simulink model "open_loop_lateral_dyn_2023b"  (R2023b)
settings: Solver=VariableStepAuto  StartTime=0.0  StopTime=Ts  RelTol=1e-3
values from neighbouring files (symbols this model uses):
  A = [0 1 0 0 ... (first row only)    [system_mat.m]
  af = 1.3    [Gain.m]    (also in Init.m; beta_vs_delta_tf.m; r_vs_delta_tf.m; system_mat.m)
  ar = 1.5    [Gain.m]    (also in Init.m; beta_vs_delta_tf.m; r_vs_delta_tf.m; system_mat.m)
  B = [B1 B2]    [system_mat.m]
  CF = 2*6*1e4    (= 120000)    [Gain.m]    (also in Init.m; beta_vs_delta_tf.m; r_vs_delta_tf.m; system_mat.m)
  CR = 2*5.7*1e4    (= 114000)    [Gain.m]    (also in Init.m; beta_vs_delta_tf.m; r_vs_delta_tf.m; system_mat.m)
  delay_return = 13+delay    (= 14)    [Init.m]
  delta_max = 25    [Gain.m]    (also in Init.m)
  dvol_drift1 = dvol_drift(1)    [Init.m]
  dvol_drift2 = dvol_drift(2)    [Init.m]
  dvol_drift3 = dvol_drift(3)    [Init.m]
  K = (m/L)*(CR*ar-(CF*af))/(CF*CR)    (= 0.000616776315789)    [Gain.m]    (also in Init.m = place(A,B(:,1),p); Poles.m = acker(A, B(:,1), P(i,:)))
  L = af+ar    (= 2.8)    [Gain.m]    (also in Init.m)
  m = 1575    [Gain.m]    (also in Init.m; beta_vs_delta_tf.m; r_vs_delta_tf.m; system_mat.m)
  sel_man = 1    [Init.m]
  t_drift_cs_1 = 5*1+3*0    (= 5)    [Init.m]
  t_drift_cs_2 = t_drift_cs_1*2    (= 10)    [Init.m]
  tau_s = 15    [Gain.m]    (also in Init.m)
  Vx = vv(i)    [Gain.m]    (also in Init.m = 22.2222222222; Transfer_functions.m = 33.3333333333)
libraries: simulink_extras x4, simulink x4
settings Model: Creator=soffy  LastModifiedBy=Martina
settings DataIOCC: ReturnWorkspaceOutputs=off

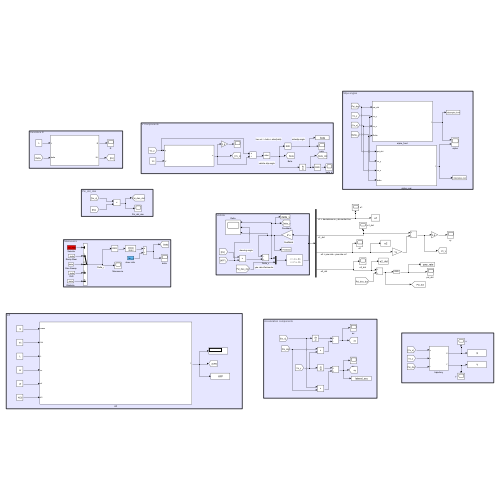
[thumbnail: Simulink's stored preview of the top-level diagram]
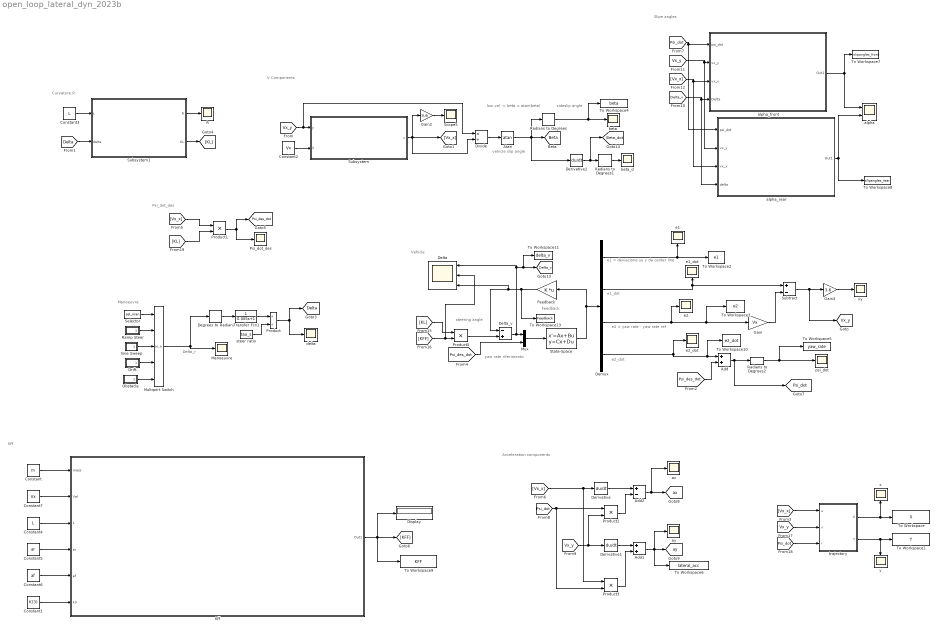
== system open_loop_lateral_dyn_2023b ==
  note: Feedback
  note: Delta_r
  note: Psi_dot_des
  note: sideslip angle
  note: Manoeuvre
  note: Vehicle
  note: Acceleration components
  note: Kff
  note: Curvature R
  note: vehicle slip angle
  note: low vel -> beta = atan(beta)
  note: V Components
  note: e2_dot
  note: e1_dot
  note: e2 = yaw rate - yaw rate ref
  note: e1 = deviazione su y da center line
  note: yaw rate riferimento
  note: steering angle
  note: Slipe angles
  Add : Sum
  Add1 : Sum
  Add2 : Sum  Inputs=+-
  Atan : Trigonometry  Operator=atan
  Constant : Constant  Value=m
  Constant1 : Constant  Value=K(3)
  Constant2 : Constant  Value=Vx
  Constant3 : Constant  Value=L
  Constant4 : Constant  Value=L
  Constant5 : Constant  Value=ar
  Constant6 : Constant  Value=af
  Constant7 : Constant  Value=Vx
  Degrees to Radians : simulink_extras/Transformations/Degrees to Radians
  Delta : Scope  NumInputPorts=3
  Delta_v : Sum  Inputs=-+
  Demux : Demux
  Derivative : Derivative
  Derivative1 : Derivative
  Derivative2 : Derivative
  Display : Display
  Divide : Product  Inputs=*/
  Drift : Subsystem
  Feedback : Gain  Gain=K  Multiplication=Matrix(K*u)
  Gain : Gain  Gain=Vx
  Gain2 : Gain  Gain=3.6
  Gain3 : Gain  Gain=3.6
  Kff : Subsystem
  Manoeuvre : Scope
  Multiport Switch : MultiPortSwitch  Inputs=4  SaturateOnIntegerOverflow=off  InputSameDT=off
  Mux : Mux  Inputs=2
  Obstacle : Subsystem
  Product : Product  Inputs=*/  RndMeth=Zero
  Product{1..3,5} (4 alike) : Product
  Psi_dot_des : Scope
  R : Scope
  Radians to Degrees : simulink_extras/Transformations/Radians to Degrees
  Radians to Degrees1 : simulink_extras/Transformations/Radians to Degrees
  Radians to Degrees2 : simulink_extras/Transformations/Radians to Degrees
  Ramp Steer : Subsystem
  Scope5 : Scope
  Selector : Constant  Value=sel_man
  Sine Sweep : Subsystem
  State-Space : StateSpace  A=A  B=B  C=eye(4)  D=zeros(4,2)  InitialCondition=0
  Subsystem : Subsystem
  Subsystem1 : Subsystem
  Subtract : Sum  Inputs=+-
  To Workspace : ToWorkspace  VariableName=X  SaveFormat=Timeseries  SampleTime=-1
  To Workspace1 : ToWorkspace  VariableName=Y  SaveFormat=Timeseries  SampleTime=-1
  To Workspace10 : ToWorkspace  VariableName=e2_dot  SaveFormat=Timeseries  SampleTime=-1
  To Workspace11 : ToWorkspace  VariableName=delta_v  SaveFormat=Timeseries  SampleTime=-1
  To Workspace13 : ToWorkspace  VariableName=Feedback  SaveFormat=Timeseries  SampleTime=-1
  To Workspace2 : ToWorkspace  VariableName=e1  SaveFormat=Timeseries  SampleTime=-1
  To Workspace3 : ToWorkspace  VariableName=e2  SaveFormat=Timeseries  SampleTime=-1
  To Workspace4 : ToWorkspace  VariableName=beta  SaveFormat=Timeseries  SampleTime=-1
  To Workspace5 : ToWorkspace  VariableName=yaw_rate  SaveFormat=Timeseries  SampleTime=-1
  To Workspace6 : ToWorkspace  VariableName=lateral_acc  SaveFormat=Timeseries  SampleTime=-1
  To Workspace7 : ToWorkspace  VariableName=slipangles_front  SaveFormat=Timeseries  SampleTime=-1
  To Workspace8 : ToWorkspace  VariableName=slipangles_rear  SaveFormat=Timeseries  SampleTime=-1
  To Workspace9 : ToWorkspace  VariableName=KFF  SaveFormat=Timeseries  SampleTime=-1
  Transfer Fcn1 : TransferFcn  Denominator=[0.005 1]
  alpha : Scope  NumInputPorts=2
  alpha_front : Subsystem
  alpha_rear : Subsystem
  ax : Scope
  ay : Scope
  beta : Scope
  beta_d : Scope
  delta : Scope
  e1 : Scope
  e1_dot : Scope
  e2 : Scope
  e2_dot : Scope
  "psi_dot " : Scope
  "steer ratio " : Constant  Value=tau_s
  trajectory : Subsystem
  vy : Scope
  x : Scope
  y : Scope
  tag scope: Beta=global, Beta_dot=global, Delta=global, Delta_v=global, Psi_des_dot=global, Psi_dot=global, Vx_y=global, ax=global, ay=global
  wires:
  Mux/1 -> State-Space/1
  State-Space/1 -> Feedback/1, Demux/1
  Demux/1 -> To Workspace2/1, e1/1
  Demux/2 -> e1_dot/1, Subtract/1
  Demux/3 -> To Workspace3/1, Gain/1, e2/1
  Demux/4 -> e2_dot/1, To Workspace10/1, Add/1
  Degrees to Radians/1 -> Transfer Fcn1/1
  Transfer Fcn1/1 -> Product/1
  "steer ratio "/1 -> Product/2
  Product/1 -> [Delta], delta/1
  Gain/1 -> Subtract/2
  Subtract/1 -> Gain3/1, [Vx_y]
  Add/1 -> [Psi_dot], Radians to Degrees2/1
  Radians to Degrees2/1 -> To Workspace5/1, "psi_dot "/1
  Subsystem/1(x) -> Gain2/1, [Vx_x], Divide/2
  [Vx_y] -> Divide/1, Subsystem/1(y)
  Constant2/1 -> Subsystem/2(V)
  Constant3/1 -> Subsystem1/1(L)
  [Delta] -> Subsystem1/2(delta)
  Subsystem1/2(KL) -> [KL]
  Kff/1(Out1) -> To Workspace9/1, Display/1, [KFF]
  Constant/1 -> Kff/1(mass)
  Constant7/1 -> Kff/2(Vel)
  Constant4/1 -> Kff/3(L)
  Constant5/1 -> Kff/4(ar)
  Constant6/1 -> Kff/5(af)
  [Psi_des_dot] -> Add/2
  [Psi_des_dot] -> Mux/2
  Divide/1 -> Atan/1
  [Vx_x] -> Product1/1
  Product1/1 -> [Psi_des_dot], Psi_dot_des/1
  Atan/1 -> Radians to Degrees/1, Derivative2/1, [Beta]
  [Vx_x] -> Product3/1, Derivative/1
  Add1/1 -> To Workspace6/1, [ay], ay/1
  [Vx_y] -> Product2/2, Derivative1/1
  Derivative1/1 -> Add1/1
  Derivative/1 -> Add2/1
  [Psi_dot] -> Product3/2, Product2/1
  Product2/1 -> Add2/2
  Product3/1 -> Add1/2
  Add2/1 -> ax/1, [ax]
  alpha_front/1(Out1) -> To Workspace7/1, alpha/1
  [Vx_x] -> alpha_rear/3(vx_x), alpha_front/3(vx_x)
  [Delta_v] -> alpha_rear/4(delta), alpha_front/4(Delta)
  [Psi_dot] -> alpha_rear/1(psi_dot), alpha_front/1(psi_dot)
  [Vx_y] -> alpha_rear/2(vx_y), alpha_front/2(vx_y)
  alpha_rear/1(Out1) -> To Workspace8/1, alpha/2
  Delta_v/1 -> To Workspace11/1, [Delta_v], Delta/1, Mux/1
  Feedback/1 -> Delta_v/1, Delta/3, To Workspace13/1
  Product5/1 -> Delta_v/2
  [KFF] -> Delta/2, Product5/2
  [KL] -> Product5/1
  Constant1/1 -> Kff/6(k3)
  Gain2/1 -> Scope5/1
  Gain3/1 -> vy/1
  Derivative2/1 -> Radians to Degrees1/1, [Beta_dot]
  [Vx_x] -> trajectory/1(u)
  [Vx_y] -> trajectory/2(v)
  trajectory/1(X) -> To Workspace/1, x/1
  trajectory/2(Y) -> To Workspace1/1, y/1
  [Psi_dot] -> trajectory/3(r)
  Radians to Degrees1/1 -> beta_d/1
  Radians to Degrees/1 -> To Workspace4/1, beta/1
  Selector/1 -> Multiport Switch/1
  Ramp Steer/1(delta) -> Multiport Switch/2
  Sine Sweep/1(delta) -> Multiport Switch/3
  Drift/1(delta) -> Multiport Switch/4
  Multiport Switch/1 -> Degrees to Radians/1, Manoeuvre/1
  [KL] -> Product1/2
  Subsystem1/1(R) -> R/1
  Obstacle/1(delta) -> Multiport Switch/5

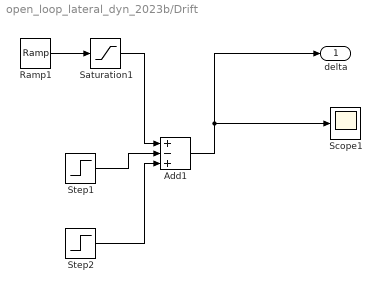
== system open_loop_lateral_dyn_2023b/Drift ==
  Add1 : Sum  Inputs=+-+
  Ramp1 : simulink/Sources/Ramp  slope=400  start=1  InitialOutput=0
  Saturation1 : Saturate  UpperLimit=dvol_drift1  LowerLimit=0
  Scope1 : Scope
  Step1 : Step  Time=t_drift_cs_1  After=dvol_drift2  SampleTime=0
  Step2 : Step  Time=t_drift_cs_2  After=dvol_drift3  SampleTime=0
  delta : Outport  VectorParamsAs1DForOutWhenUnconnected=off
  wires:
  Step2/1 -> Add1/3
  Saturation1/1 -> Add1/1
  Add1/1 -> delta/1, Scope1/1
  Step1/1 -> Add1/2
  Ramp1/1 -> Saturation1/1

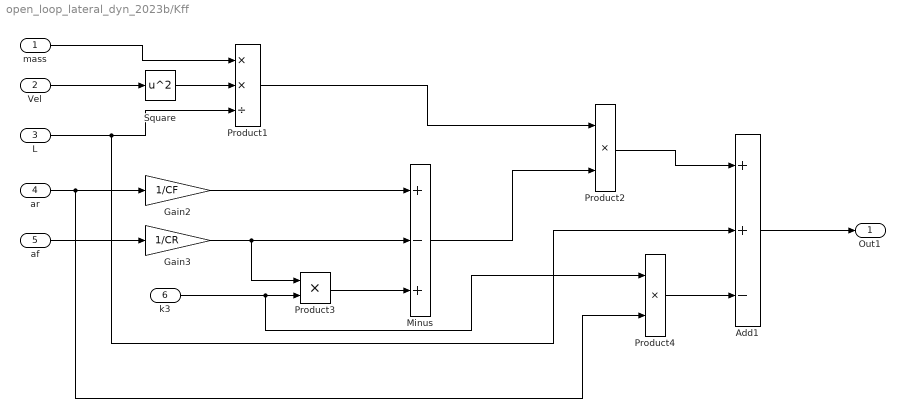
== system open_loop_lateral_dyn_2023b/Kff ==
  mass : Inport
  Vel : Inport  Port=2
  L : Inport  Port=3
  ar : Inport  Port=4
  af : Inport  Port=5
  k3 : Inport  Port=6
  Add1 : Sum  Inputs=++-
  Gain2 : Gain  Gain=1/CF
  Gain3 : Gain  Gain=1/CR
  Minus : Sum  Inputs=+-+
  Product1 : Product  Inputs=**/
  Product2 : Product
  Product3 : Product
  Product4 : Product
  Square : Math  Operator=square
  Out1 : Outport
  wires:
  Product1/1 -> Product2/1
  Product2/1 -> Add1/1
  Gain3/1 -> Minus/2, Product3/1
  Square/1 -> Product1/2
  Product4/1 -> Add1/3
  Product3/1 -> Minus/3
  k3/1 -> Product4/1, Product3/2
  Minus/1 -> Product2/2
  L/1 -> Add1/2, Product1/3
  ar/1 -> Gain2/1, Product4/2
  Gain2/1 -> Minus/1
  mass/1 -> Product1/1
  Vel/1 -> Square/1
  Add1/1 -> Out1/1
  af/1 -> Gain3/1

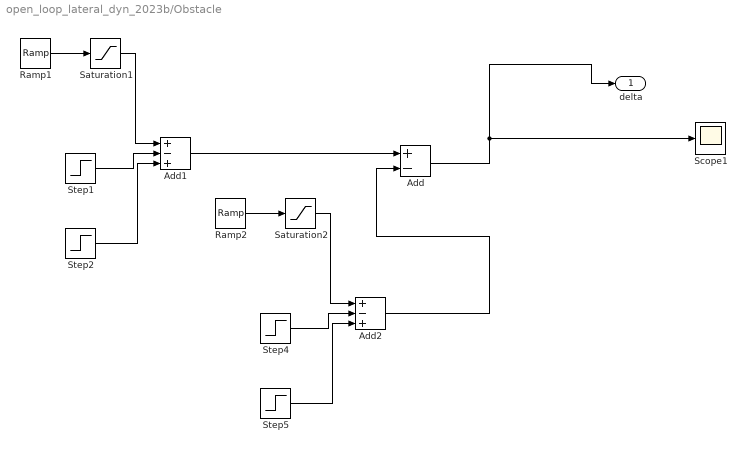
== system open_loop_lateral_dyn_2023b/Obstacle ==
  Add : Sum  Inputs=+-
  Add1 : Sum  Inputs=+-+
  Add2 : Sum  Inputs=+-+
  Ramp1 : simulink/Sources/Ramp  slope=400  start=1  InitialOutput=0
  Ramp2 : simulink/Sources/Ramp  slope=400  start=delay_return  InitialOutput=0
  Saturation1 : Saturate  UpperLimit=dvol_drift1  LowerLimit=0
  Saturation2 : Saturate  UpperLimit=dvol_drift1  LowerLimit=0
  Scope1 : Scope
  Step1 : Step  Time=t_drift_cs_1+1  After=dvol_drift1*2  SampleTime=0
  Step2 : Step  Time=t_drift_cs_1*2+1  After=dvol_drift1  SampleTime=0
  Step4 : Step  Time=t_drift_cs_1+delay_return  After=dvol_drift1*2  SampleTime=0
  Step5 : Step  Time=t_drift_cs_1*2+delay_return  After=dvol_drift1  SampleTime=0
  delta : Outport  VectorParamsAs1DForOutWhenUnconnected=off
  wires:
  Step2/1 -> Add1/3
  Saturation1/1 -> Add1/1
  Step1/1 -> Add1/2
  Ramp1/1 -> Saturation1/1
  Add1/1 -> Add/1
  Ramp2/1 -> Saturation2/1
  Saturation2/1 -> Add2/1
  Step5/1 -> Add2/3
  Step4/1 -> Add2/2
  Add/1 -> Scope1/1, delta/1
  Add2/1 -> Add/2

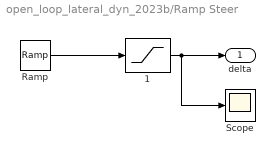
== system open_loop_lateral_dyn_2023b/Ramp Steer ==
  "  1" : Saturate  UpperLimit=delta_max  LowerLimit=0
  Ramp : simulink/Sources/Ramp  slope=400  start=1+0.01  InitialOutput=0
  Scope : Scope
  delta : Outport  VectorParamsAs1DForOutWhenUnconnected=off
  wires:
  "  1"/1 -> Scope/1, delta/1
  Ramp/1 -> "  1"/1

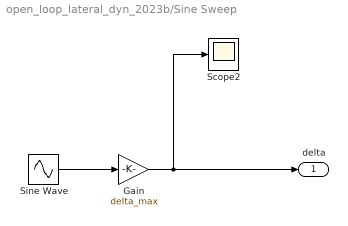
== system open_loop_lateral_dyn_2023b/Sine Sweep ==
  Gain : Gain  Gain=delta_max
  Scope2 : Scope
  Sine Wave : Sin  Amplitude=0.7  Frequency=0.5  SampleTime=0
  delta : Outport  InitialOutput=0  VectorParamsAs1DForOutWhenUnconnected=off
  wires:
  Sine Wave/1 -> Gain/1
  Gain/1 -> delta/1, Scope2/1

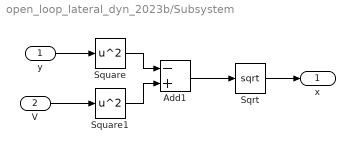
== system open_loop_lateral_dyn_2023b/Subsystem ==
  y : Inport
  V : Inport  Port=2
  Add1 : Sum  Inputs=-+
  Sqrt : Sqrt
  Square : Math  Operator=square
  Square1 : Math  Operator=square
  x : Outport
  wires:
  V/1 -> Square1/1
  Square1/1 -> Add1/2
  Add1/1 -> Sqrt/1
  Square/1 -> Add1/1
  Sqrt/1 -> x/1
  y/1 -> Square/1

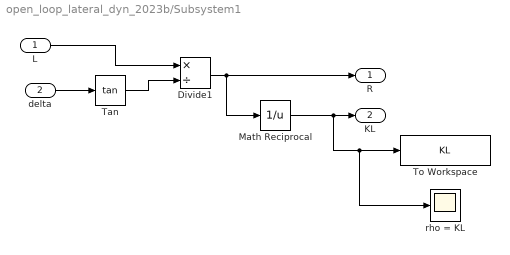
== system open_loop_lateral_dyn_2023b/Subsystem1 ==
  L : Inport
  delta : Inport  Port=2
  Divide1 : Product  Inputs=*/
  Math Reciprocal : Math  Operator=reciprocal  SignedPower=on
  Tan : Trigonometry  Operator=tan
  To Workspace : ToWorkspace  VariableName=KL  SaveFormat=Timeseries  SampleTime=-1
  rho = KL : Scope
  R : Outport
  KL : Outport  Port=2
  wires:
  Tan/1 -> Divide1/2
  Divide1/1 -> R/1, Math Reciprocal/1
  L/1 -> Divide1/1
  delta/1 -> Tan/1
  Math Reciprocal/1 -> rho = KL/1, To Workspace/1, KL/1

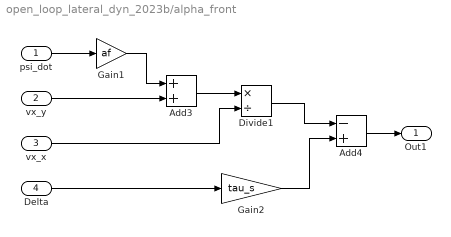
== system open_loop_lateral_dyn_2023b/alpha_front ==
  psi_dot : Inport
  vx_y : Inport  Port=2
  vx_x : Inport  Port=3
  Delta : Inport  Port=4
  Add3 : Sum
  Add4 : Sum  Inputs=-+
  Divide1 : Product  Inputs=*/
  Gain1 : Gain  Gain=af
  Gain2 : Gain  Gain=tau_s
  Out1 : Outport
  wires:
  Add3/1 -> Divide1/1
  vx_y/1 -> Add3/2
  Gain2/1 -> Add4/2
  Gain1/1 -> Add3/1
  psi_dot/1 -> Gain1/1
  Divide1/1 -> Add4/1
  Add4/1 -> Out1/1
  vx_x/1 -> Divide1/2
  Delta/1 -> Gain2/1

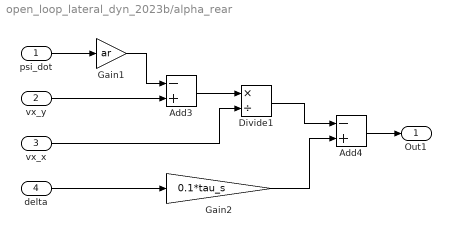
== system open_loop_lateral_dyn_2023b/alpha_rear ==
  psi_dot : Inport
  vx_y : Inport  Port=2
  vx_x : Inport  Port=3
  delta : Inport  Port=4
  Add3 : Sum  Inputs=-+
  Add4 : Sum  Inputs=-+
  Divide1 : Product  Inputs=*/
  Gain1 : Gain  Gain=ar
  Gain2 : Gain  Gain=0.1*tau_s
  Out1 : Outport
  wires:
  Add3/1 -> Divide1/1
  vx_y/1 -> Add3/2
  Gain2/1 -> Add4/2
  Gain1/1 -> Add3/1
  psi_dot/1 -> Gain1/1
  Divide1/1 -> Add4/1
  Add4/1 -> Out1/1
  vx_x/1 -> Divide1/2
  delta/1 -> Gain2/1

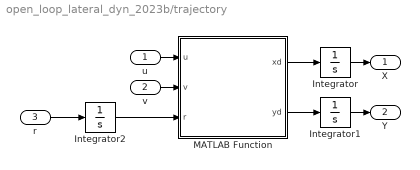
== system open_loop_lateral_dyn_2023b/trajectory ==
  u : Inport
  v : Inport  Port=2
  r : Inport  Port=3
  Integrator : Integrator
  Integrator1 : Integrator
  Integrator2 : Integrator
  MATLAB Function : MATLAB Function  TreatAsAtomicUnit=on
  X : Outport
  Y : Outport  Port=2
  wires:
  Integrator1/1 -> Y/1
  MATLAB Function/2(yd) -> Integrator1/1
  r/1 -> Integrator2/1
  MATLAB Function/1(xd) -> Integrator/1
  u/1 -> MATLAB Function/1(u)
  Integrator/1 -> X/1
  v/1 -> MATLAB Function/2(v)
  Integrator2/1 -> MATLAB Function/3(r)

== matlab function open_loop_lateral_dyn_2023b/trajectory/MATLAB Function ==
  data: u input; xd output; v input; r input; yd output
function [xd, yd] = trajectory(u, v, r)

xd = u*cos(r)- (v*sin(r));
yd = v*cos(r) + (u*sin(r));

end
